simulink model "integral_discrete_control"  (R2016a)
settings: Solver=VariableStepAuto  StartTime=0.0  StopTime=.04  RelTol=1e-4
values from neighbouring files (symbols this model uses):
  K = place(A,B,P)    [calculate_gains.m]
  K1 = K_i(1:2)    [calculate_gains.m]
  K1_d = K_d(1:2)    [calculate_gains.m]
  K2 = K_i(3)    [calculate_gains.m]
  K2_d = K_d(3)    [calculate_gains.m]
  Ts = 4e-4    (= 0.0004)    [calculate_gains.m]    (also in generate_lookup_table.m = 0.0005)
undefined symbols (not defined in the file or in its folder): DiscIntNeverNeededParam
settings Model: Creator=manuel  LastModifiedBy=manuel

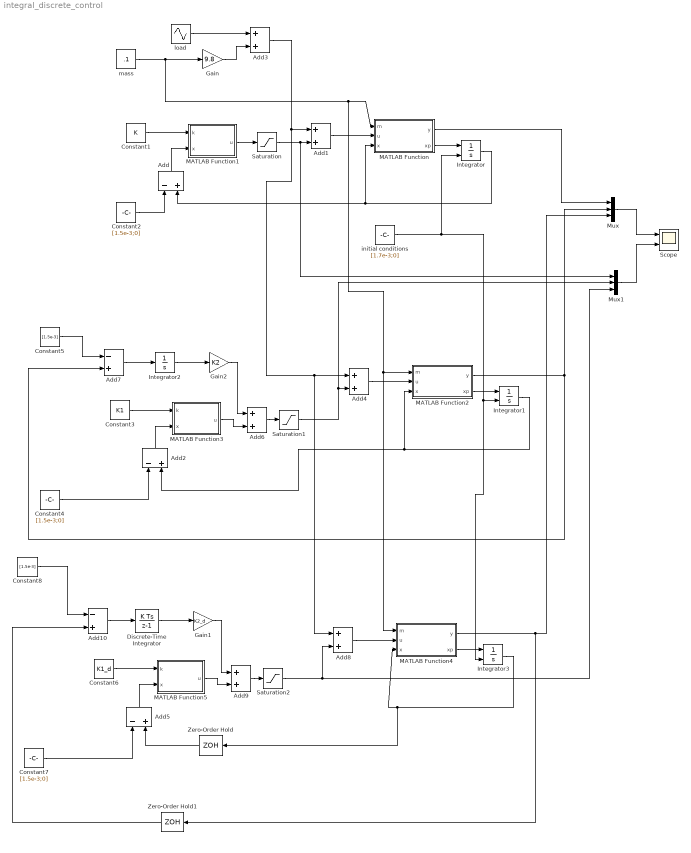
== system integral_discrete_control ==
  Add{,2,5,7,10} (5 alike) : Sum  Inputs=-+
  Add{1,3..4,6,8..9} (6 alike) : Sum
  Constant1 : Constant  Value=K
  Constant2 : Constant  Value=[1.5e-3;0]
  Constant3 : Constant  Value=K1
  Constant4 : Constant  Value=[1.5e-3;0]
  Constant5 : Constant  Value=[1.5e-3]
  Constant6 : Constant  Value=K1_d
  Constant7 : Constant  Value=[1.5e-3;0]
  Constant8 : Constant  Value=[1.5e-3]
  Discrete-Time Integrator : DiscreteIntegrator  InitialConditionSetting=State (most efficient)  SampleTime=Ts  ICPrevOutput=DiscIntNeverNeededParam  ICPrevScaledInput=DiscIntNeverNeededParam
  Gain : Gain  Gain=9.8
  Gain1 : Gain  Gain=K2_d
  Gain2 : Gain  Gain=K2
  Integrator : Integrator  InitialConditionSource=external  InitialCondition=[1.6e-3;0]  LimitOutput=on  UpperSaturationLimit=[2e-3;inf]  LowerSaturationLimit=[1e-3;-inf]
  Integrator1 : Integrator  InitialConditionSource=external  InitialCondition=[1.6e-3;0]  LimitOutput=on  UpperSaturationLimit=[2e-3;inf]  LowerSaturationLimit=[1e-3;-inf]
  Integrator2 : Integrator  InitialCondition=[0]  UpperSaturationLimit=[2e-3;inf]  LowerSaturationLimit=[1e-3;-inf]
  Integrator3 : Integrator  InitialConditionSource=external  InitialCondition=[1.6e-3;0]  LimitOutput=on  UpperSaturationLimit=[2e-3;inf]  LowerSaturationLimit=[1e-3;-inf]
  MATLAB Function : MATLAB Function  TreatAsAtomicUnit=on
  MATLAB Function1 : MATLAB Function  TreatAsAtomicUnit=on
  MATLAB Function2 : MATLAB Function  TreatAsAtomicUnit=on
  MATLAB Function3 : MATLAB Function  TreatAsAtomicUnit=on
  MATLAB Function4 : MATLAB Function  TreatAsAtomicUnit=on
  MATLAB Function5 : MATLAB Function  TreatAsAtomicUnit=on
  Mux : Mux  Inputs=3
  Mux1 : Mux  Inputs=3
  Saturation : Saturate  UpperLimit=9.8  LowerLimit=-9.8
  Saturation1 : Saturate  UpperLimit=9.8  LowerLimit=-9.8
  Saturation2 : Saturate  UpperLimit=9.8  LowerLimit=-9.8
  Scope : Scope  NumInputPorts=2
  Zero-Order Hold : ZeroOrderHold  SampleTime=Ts
  Zero-Order Hold1 : ZeroOrderHold  SampleTime=Ts
  initial conditions : Constant  Value=[1.7e-3;0]
  load : Sin  Bias=1  Frequency=2*pi*100  SampleTime=0
  mass : Constant  Value=.1
  wires:
  MATLAB Function/2(xp) -> Integrator/1
  Integrator/1 -> MATLAB Function/3(x), Add/2
  MATLAB Function/1(y) -> Mux/1
  Constant1/1 -> MATLAB Function1/1(k)
  Constant2/1 -> Add/1
  Add/1 -> MATLAB Function1/2(x)
  Add1/1 -> MATLAB Function/2(u)
  Gain/1 -> Add3/2
  load/1 -> Add3/1
  Mux/1 -> Scope/1
  Mux1/1 -> Scope/2
  MATLAB Function1/1(u) -> Saturation/1
  Saturation/1 -> Mux1/1, Add1/2
  MATLAB Function2/2(xp) -> Integrator1/1
  Integrator1/1 -> Add2/2, MATLAB Function2/3(x)
  MATLAB Function2/1(y) -> Add7/2, Mux/2
  Constant3/1 -> MATLAB Function3/1(k)
  Constant4/1 -> Add2/1
  Add2/1 -> MATLAB Function3/2(x)
  Add4/1 -> MATLAB Function2/2(u)
  Saturation1/1 -> Mux1/2, Add4/2
  Integrator2/1 -> Gain2/1
  Add6/1 -> Saturation1/1
  Gain2/1 -> Add6/1
  MATLAB Function3/1(u) -> Add6/2
  Add7/1 -> Integrator2/1
  Constant5/1 -> Add7/1
  MATLAB Function4/2(xp) -> Integrator3/1
  Integrator3/1 -> Zero-Order Hold/1, MATLAB Function4/3(x)
  Constant6/1 -> MATLAB Function5/1(k)
  Constant7/1 -> Add5/1
  Add5/1 -> MATLAB Function5/2(x)
  Add8/1 -> MATLAB Function4/2(u)
  Add3/1 -> Add4/1, Add8/1, Add1/1
  initial conditions/1 -> Integrator3/2, Integrator1/2, Integrator/2
  Saturation2/1 -> Mux1/3, Add8/2
  Add9/1 -> Saturation2/1
  Gain1/1 -> Add9/1
  MATLAB Function5/1(u) -> Add9/2
  Constant8/1 -> Add10/1
  mass/1 -> Gain/1, MATLAB Function4/1(m), MATLAB Function2/1(m), MATLAB Function/1(m)
  Zero-Order Hold/1 -> Add5/2
  MATLAB Function4/1(y) -> Zero-Order Hold1/1, Mux/3
  Add10/1 -> Discrete-Time Integrator/1
  Zero-Order Hold1/1 -> Add10/2
  Discrete-Time Integrator/1 -> Gain1/1

== matlab function integral_discrete_control/MATLAB Function1 ==
  data: k input; x input; u output
function u = fcn(k,x)
%#codegen

u = -k'*x;

== matlab function integral_discrete_control/MATLAB Function ==
  data: m input; u input; x input; y output; xp output
function [y,xp] = mass_model(m,u,x)
%#codegen
A = [0 1
     0 0];
B = [0;
     1/m];
C = [1 0];

xp = A*x + B*u;
y = C*x;

== matlab function integral_discrete_control/MATLAB Function2 ==
  data: m input; u input; x input; y output; xp output
function [y,xp] = mass_model(m,u,x)
%#codegen
A = [0 1
     0 0];
B = [0;
     1/m];
C = [1 0];

xp = A*x + B*u;
y = C*x;

== matlab function integral_discrete_control/MATLAB Function3 ==
  data: k input; x input; u output
function u = fcn(k,x)
%#codegen

u = -k'*x;

== matlab function integral_discrete_control/MATLAB Function4 ==
  data: m input; u input; x input; y output; xp output
function [y,xp] = mass_model(m,u,x)
%#codegen
A = [0 1
     0 0];
B = [0;
     1/m];
C = [1 0];

xp = A*x + B*u;
y = C*x;

== matlab function integral_discrete_control/MATLAB Function5 ==
  data: k input; x input; u output
function u = fcn(k,x)
%#codegen

u = -k'*x;
